simulink library "sixDoF_ul"  (R2020a)
settings: Solver=VariableStepAuto  StartTime=0.0  StopTime=10.0  RelTol=1e-3
undefined symbols (not defined in the file): init_Euler, init_O_rKite, init_O_vKite, init_OwB
libraries: vrlib x1, eulDot x1, makeOcB_cl x1
settings Model: Creator=Ayaz  LastModifiedBy=Ayaz

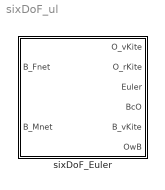
== system sixDoF_ul ==
  sixDoF_Euler : Subsystem  mask{mass=36.8, Jmat=eye(3), init_O_vKite=init_O_vKite, init_O_rKite=init_O_rKite, init_OwB=init_OwB, init_Euler=init_Euler}
      mask prompts: mass "Mass [kg]"; Jmat "Inertial [kj-m^2]"; init_O_vKite "Initial inertial velocity [m/s]"; init_O_rKite "Initial inertial position [m]"; init_OwB "Initial angular velocity [rad/s]"; init_Euler "Initial Euler angles [rad]"
      mask init:
      | invJmat = inv(Jmat);
      mask TypeOptions mass: Constant/Value
      mask TypeOptions Jmat: Constant1/Value
      mask TypeOptions init_O_vKite: Integrator/InitialCondition
      mask TypeOptions init_O_rKite: Integrator1/InitialCondition
      mask TypeOptions init_OwB: Integrator2/InitialCondition
      mask TypeOptions init_Euler: Integrator3/InitialCondition

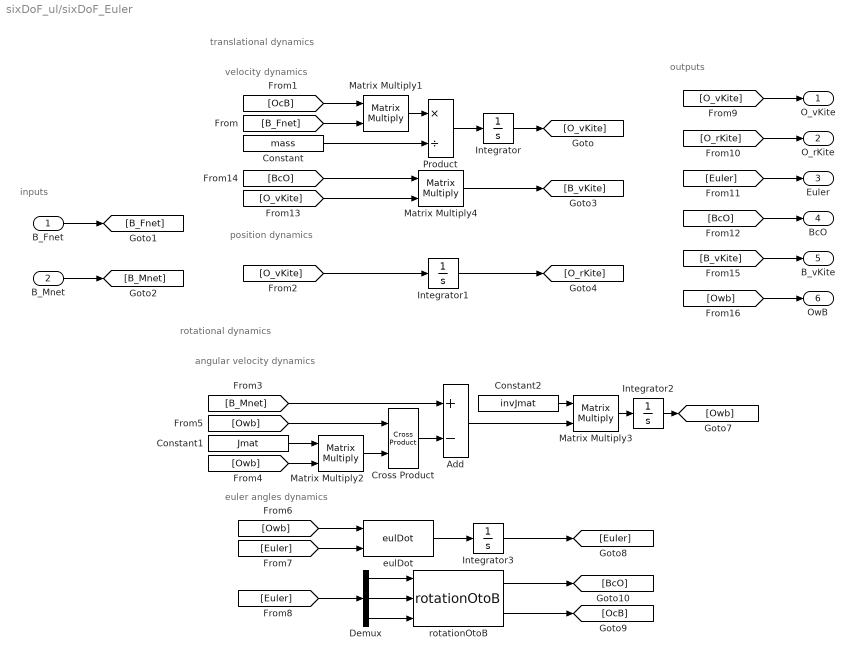
== system sixDoF_ul/sixDoF_Euler ==
  note: outputs
  note: translational dynamics
  note: position dynamics
  note: velocity dynamics
  note: rotational dynamics
  note: angular velocity dynamics
  note: euler angles dynamics
  note: inputs
  B_Fnet : Inport
  B_Mnet : Inport  Port=2
  Add : Sum  Inputs=+-
  Constant : Constant  Value=mass
  Constant1 : Constant  Value=Jmat  VectorParams1D=off
  Constant2 : Constant  Value=invJmat  VectorParams1D=off
  Cross Product : vrlib/Utilities/Cross Product
  Demux : Demux  Outputs=3
  Integrator : Integrator  InitialCondition=init_O_vKite
  Integrator1 : Integrator  InitialCondition=init_O_rKite
  Integrator2 : Integrator  InitialCondition=init_OwB
  Integrator3 : Integrator  InitialCondition=init_Euler
  Matrix Multiply{1..4} (4 alike) : Product  Multiplication=Matrix(*)
  Product : Product  Inputs=*/
  eulDot : eulDot/eulDot  SystemSampleTime=-1  Latency=0  AutoFrameSizeCalculation=off
  rotationOtoB : makeOcB_cl/rotationOtoB  SystemSampleTime=-1  Latency=0  AutoFrameSizeCalculation=off
  O_vKite : Outport
  O_rKite : Outport  Port=2
  Euler : Outport  Port=3
  BcO : Outport  Port=4
  B_vKite : Outport  Port=5
  OwB : Outport  Port=6
  wires:
  B_Fnet/1 -> [B_Fnet]
  B_Mnet/1 -> [B_Mnet]
  Constant/1 -> Product/2
  Integrator/1 -> [O_vKite]
  [B_Fnet] -> Matrix Multiply1/2
  [OcB] -> Matrix Multiply1/1
  Matrix Multiply1/1 -> Product/1
  Product/1 -> Integrator/1
  [O_vKite] -> Integrator1/1
  Integrator1/1 -> [O_rKite]
  Constant1/1 -> Matrix Multiply2/1
  [Owb] -> Matrix Multiply2/2
  Matrix Multiply2/1 -> Cross Product/2
  [Owb] -> Cross Product/1
  Cross Product/1 -> Add/2
  [B_Mnet] -> Add/1
  Add/1 -> Matrix Multiply3/2
  Constant2/1 -> Matrix Multiply3/1
  Matrix Multiply3/1 -> Integrator2/1
  Integrator2/1 -> [Owb]
  [Owb] -> eulDot/1
  [Euler] -> eulDot/2
  eulDot/1 -> Integrator3/1
  Integrator3/1 -> [Euler]
  Demux/1 -> rotationOtoB/1
  Demux/2 -> rotationOtoB/2
  Demux/3 -> rotationOtoB/3
  [Euler] -> Demux/1
  rotationOtoB/2 -> [OcB]
  rotationOtoB/1 -> [BcO]
  [O_vKite] -> O_vKite/1
  [O_rKite] -> O_rKite/1
  [Euler] -> Euler/1
  [BcO] -> BcO/1
  [O_vKite] -> Matrix Multiply4/2
  [BcO] -> Matrix Multiply4/1
  Matrix Multiply4/1 -> [B_vKite]
  [B_vKite] -> B_vKite/1
  [Owb] -> OwB/1
